simulink model "throttle_control"  (R2021a)
settings: Solver=FixedStepAuto  StartTime=0.0  StopTime=inf  FixedStep=1/2000  RelTol=1e-3
undefined symbols (not defined in the file): Brake, Steer, Throttle
libraries: robotlib x5, pid_lib x2
settings Model: Creator=refulgent  LastModifiedBy=refulgent
settings OptimizationCC: EnhancedBackFolding=on  PassReuseOutputArgsAs=Individual arguments  ZeroExternalMemoryAtStartup=off  ZeroInternalMemoryAtStartup=off  MaxStackSize=64  OptimizeBlockOrder=speed  DifferentSizesBufferReuse=on  EfficientTunableParamExpr=on
settings DebuggingCC: ParameterTunabilityLossMsg=error
settings HardwareCC: ProdBitPerPointer=32  ProdBitPerSizeT=32  ProdBitPerPtrDiffT=32  ProdLargestAtomicFloat=None  ProdIntDivRoundTo=Undefined  ProdEndianess=Unspecified  ProdWordSize=32  ProdHWDeviceType=Generic->Unspecified (assume 32-bit Generic)
settings SFSimCC: MATLABDynamicMemAlloc=off
settings RTWCC: SystemTargetFile=ert.tlc  HardwareBoard=Robot Operating System (ROS)  TLCOptions="-aInlineSetEventsForThisBaseRateFcn=TLC_FALSE -aSuppressMultiTaskScheduler=TLC_FALSE  -aRateBasedStepFcn=0"  TemplateMakefile=ert_default_tmf  Toolchain=Catkin  TargetLang=C++
settings CodeAppCC: ForceParamTrailComments=on  IgnoreCustomStorageClasses=off  OperatorAnnotations=on  SimulinkDataObjDesc=on  SFDataObjDesc=on  InsertBlockDesc=on
settings ERTTargetCC: SupportContinuousTime=on

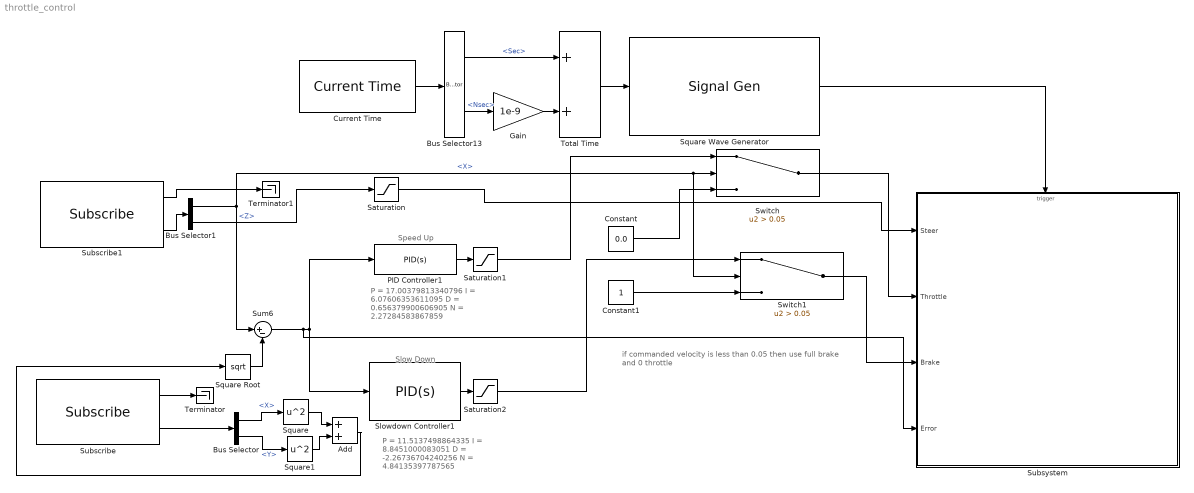
== system throttle_control ==
  note: if commanded velocity is less than 0.05 then use full brake
      | and 0 throttle
  note: P = 17.00379813340796
      | I = 6.07606353611095
      | D = 0.656379900606905
      | N = 2.27284583867859
  note: Slow Down
  note: Speed Up
  note: P = 11.5137498864335
      | I = 8.8451000083051
      | D = -2.26736704240256
      | N = 4.84135397787565
  Add : Sum
  Bus Selector : BusSelector  OutputSignals=Linear.X,Linear.Y
  Bus Selector1 : BusSelector  OutputSignals=Linear.X,Angular.Z
  Bus Selector13 : BusSelector  OutputSignals=Sec,Nsec
  Constant : Constant  Value=0.0
  Constant1 : Constant
  Current Time : robotlib/Current Time  OutputFormat=bus  SampleTime=-1  ModelName=throttle_control
      settings: SourceProductBaseCode=RR
  Gain : Gain  Gain=1e-9
  PID Controller1 : pid_lib/PID Controller  Controller=PID  Form=Parallel  TimeDomain=Continuous-time  UseExternalTs=off  SampleTime=-1  IntegratorMethod=Forward Euler  FilterMethod=Forward Euler  ControllerParametersSource=internal  P=17.00379813340796  I=6.07606353611095  D=0.656379900606905  UseFilter=on  N=2.27284583867859  TunerSelectOption=Transfer Function Based (PID Tuner App)  InitialConditionSource=internal  InitialConditionForIntegrator=0  InitialConditionForFilter=0  DifferentiatorICPrevScaledInput=0  ExternalReset=none  TrackingMode=off  Kt=1  LimitOutput=on  SatLimitsSource=internal  UpperSaturationLimit=1  LowerSaturationLimit=0  LinearizeAsGain=on  AntiWindupMode=clamping  Kb=1  POutMin=[]  POutMax=[]  IOutMin=[]  IOutMax=[]  DOutMin=[]  DOutMax=[]  NOutMin=[]  NOutMax=[]  SumOutMin=[]  SumOutMax=[]  SaturationOutMin=[]  SaturationOutMax=[]  PParamMin=[]  PParamMax=[]  IParamMin=[]  IParamMax=[]  DParamMin=[]  DParamMax=[]  NParamMin=[]  NParamMax=[]  KbParamMin=[]  KbParamMax=[]  KtParamMin=[]  KtParamMax=[]  KbOutMin=[]  KbOutMax=[]  KtOutMin=[]  KtOutMax=[]  IntegratorOutMin=[]  IntegratorOutMax=[]  FilterOutMin=[]  FilterOutMax=[]  SumI1OutMin=[]  SumI1OutMax=[]  SumI2OutMin=[]  SumI2OutMax=[]  SumI3OutMin=[]  SumI3OutMax=[]  SumI4OutMin=[]  SumI4OutMax=[]  SumDOutMin=[]  SumDOutMax=[]  DifferentiatorOutMin=[]  DifferentiatorOutMax=[]  FilterDiffOutCoefMin=[]  FilterDiffOutCoefMax=[]  ReciprocalOutMin=[]  ReciprocalOutMax=[]  SumDenOutMin=[]  SumDenOutMax=[]  SumNumOutMin=[]  SumNumOutMax=[]  DivideOutMin=[]  DivideOutMax=[]  UdiffTsProdOutMin=[]  UdiffTsProdOutMax=[]  NTsProdOutMin=[]  NTsProdOutMax=[]  UintegralTsProdOutMin=[]  UintegralTsProdOutMax=[]  UngainTsProdOutMin=[]  UngainTsProdOutMax=[]  IntegratorContinuousStateAttributes=''  IntegratorStateMustResolveToSignalObject=off  IntegratorRTWStateStorageClass=Auto  FilterContinuousStateAttributes=''  FilterStateMustResolveToSignalObject=off  FilterRTWStateStorageClass=Auto  ParallelPVariant=InternalParameters  IdealPVariant=Disabled  IVariant=InternalParameters  DVariant=InternalParameters  IntegratorVariant=Continuous  SatVariant=Enabled  AWVariant=ContClampingParallel  PCopyVariant=Disabled  TRVariant=Disabled  FdbkBlocksVariant=Forward  IdealPFdbkVariant=Disabled  SatFdbkVariant=Disabled  DerivativeFilterVariant=ContFilter  NVariant=InternalParameters  NCopyVariant=Disabled  FilterICVariant=InternalICsFilter  IntegratorICVariant=InternalICs  ExternalResetVariant=Disabled  TRSumVariant=Passthrough  SumFdbkVariant=Disabled  SumVariant=Sum_PID  TsampFilterVariant=InternalTs  TsampNgainVariant=Passthrough  TsampIntegralVariant=Passthrough  ExternalSaturationOutDataTypeStr=Inherit: Same as second input
  Saturation : Saturate  UpperLimit=1  LowerLimit=-1
  Saturation1 : Saturate  UpperLimit=1  LowerLimit=0
  Saturation2 : Saturate  UpperLimit=1  LowerLimit=0
  Slowdown Controller1 : pid_lib/PID Controller  Controller=PID  Form=Parallel  TimeDomain=Continuous-time  UseExternalTs=off  SampleTime=-1  IntegratorMethod=Forward Euler  FilterMethod=Forward Euler  ControllerParametersSource=internal  P=11.5137498864335  I=8.8451000083051  D=-2.26736704240256  UseFilter=on  N=4.84135397787565  TunerSelectOption=Transfer Function Based (PID Tuner App)  InitialConditionSource=internal  InitialConditionForIntegrator=0  InitialConditionForFilter=0  DifferentiatorICPrevScaledInput=0  ExternalReset=none  TrackingMode=off  Kt=1  LimitOutput=on  SatLimitsSource=internal  UpperSaturationLimit=1  LowerSaturationLimit=0  LinearizeAsGain=on  AntiWindupMode=clamping  Kb=1  POutMin=[]  POutMax=[]  IOutMin=[]  IOutMax=[]  DOutMin=[]  DOutMax=[]  NOutMin=[]  NOutMax=[]  SumOutMin=[]  SumOutMax=[]  SaturationOutMin=[]  SaturationOutMax=[]  PParamMin=[]  PParamMax=[]  IParamMin=[]  IParamMax=[]  DParamMin=[]  DParamMax=[]  NParamMin=[]  NParamMax=[]  KbParamMin=[]  KbParamMax=[]  KtParamMin=[]  KtParamMax=[]  KbOutMin=[]  KbOutMax=[]  KtOutMin=[]  KtOutMax=[]  IntegratorOutMin=[]  IntegratorOutMax=[]  FilterOutMin=[]  FilterOutMax=[]  SumI1OutMin=[]  SumI1OutMax=[]  SumI2OutMin=[]  SumI2OutMax=[]  SumI3OutMin=[]  SumI3OutMax=[]  SumI4OutMin=[]  SumI4OutMax=[]  SumDOutMin=[]  SumDOutMax=[]  DifferentiatorOutMin=[]  DifferentiatorOutMax=[]  FilterDiffOutCoefMin=[]  FilterDiffOutCoefMax=[]  ReciprocalOutMin=[]  ReciprocalOutMax=[]  SumDenOutMin=[]  SumDenOutMax=[]  SumNumOutMin=[]  SumNumOutMax=[]  DivideOutMin=[]  DivideOutMax=[]  UdiffTsProdOutMin=[]  UdiffTsProdOutMax=[]  NTsProdOutMin=[]  NTsProdOutMax=[]  UintegralTsProdOutMin=[]  UintegralTsProdOutMax=[]  UngainTsProdOutMin=[]  UngainTsProdOutMax=[]  IntegratorContinuousStateAttributes=''  IntegratorStateMustResolveToSignalObject=off  IntegratorRTWStateStorageClass=Auto  FilterContinuousStateAttributes=''  FilterStateMustResolveToSignalObject=off  FilterRTWStateStorageClass=Auto  ParallelPVariant=InternalParameters  IdealPVariant=Disabled  IVariant=InternalParameters  DVariant=InternalParameters  IntegratorVariant=Continuous  SatVariant=Enabled  AWVariant=ContClampingParallel  PCopyVariant=Disabled  TRVariant=Disabled  FdbkBlocksVariant=Forward  IdealPFdbkVariant=Disabled  SatFdbkVariant=Disabled  DerivativeFilterVariant=ContFilter  NVariant=InternalParameters  NCopyVariant=Disabled  FilterICVariant=InternalICsFilter  IntegratorICVariant=InternalICs  ExternalResetVariant=Disabled  TRSumVariant=Passthrough  SumFdbkVariant=Disabled  SumVariant=Sum_PID  TsampFilterVariant=InternalTs  TsampNgainVariant=Passthrough  TsampIntegralVariant=Passthrough  ExternalSaturationOutDataTypeStr=Inherit: Same as second input
  Square : Math  Operator=square  SaturateOnIntegerOverflow=on
  Square Root : Sqrt  SaturateOnIntegerOverflow=on
  Square Wave Generator : SignalGenerator  WaveForm=square  TimeSource=Use external signal  Frequency=100
  Square1 : Math  Operator=square  SaturateOnIntegerOverflow=on
  Subscribe : robotlib/Subscribe  topicSource=Specify your own  topic=vel  messageType=geometry_msgs/Twist  SampleTime=-1  legacyBusStruct=off  messageQueueLength=1
  Subscribe1 : robotlib/Subscribe  topicSource=Specify your own  topic=cmd_vel  messageType=geometry_msgs/Twist  SampleTime=-1  legacyBusStruct=off  messageQueueLength=1
  Subsystem : Subsystem
  Sum6 : Sum  Inputs=|+-
  Switch : Switch  Criteria=u2 > Threshold  Threshold=0.05
  Switch1 : Switch  Criteria=u2 > Threshold  Threshold=0.05
  Terminator : Terminator
  Terminator1 : Terminator
  Total Time : Sum
  wires:
  Sum6/1 -> Subsystem/4(Error), Slowdown Controller1/1, PID Controller1/1
  Subscribe/2 -> Bus Selector/1
  Bus Selector/1 -> Square/1  "<X>"
  Bus Selector/2 -> Square1/1  "<Y>"
  Square1/1 -> Add/2
  Square/1 -> Add/1
  Add/1 -> Square Root/1
  Square Root/1 -> Sum6/2
  Subscribe/1 -> Terminator/1
  Subscribe1/1 -> Terminator1/1
  Subscribe1/2 -> Bus Selector1/1
  Bus Selector1/1 -> Sum6/1, Switch1/2, Switch/2  "<X>"
  Bus Selector1/2 -> Saturation/1  "<Z>"
  Saturation/1 -> Subsystem/1(Steer)
  Saturation1/1 -> Switch/1
  Slowdown Controller1/1 -> Saturation2/1
  Bus Selector13/1 -> Total Time/1  "<Sec>"
  Square Wave Generator/1 -> Subsystem/Trigger
  Bus Selector13/2 -> Gain/1  "<Nsec>"
  Total Time/1 -> Square Wave Generator/1
  Gain/1 -> Total Time/2
  Current Time/1 -> Bus Selector13/1
  PID Controller1/1 -> Saturation1/1
  Saturation2/1 -> Switch1/1
  Constant/1 -> Switch/3
  Switch/1 -> Subsystem/2(Throttle)
  Constant1/1 -> Switch1/3
  Switch1/1 -> Subsystem/3(Brake)

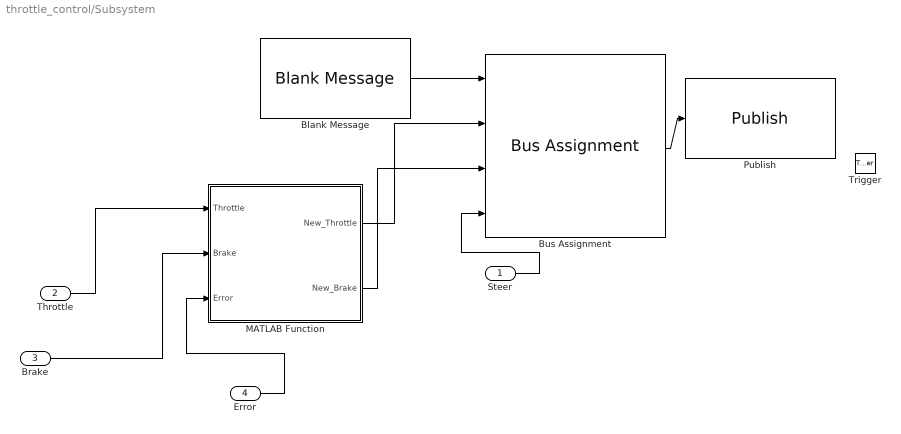
== system throttle_control/Subsystem ==
  Steer : Inport
  Throttle : Inport  Port=2
  Brake : Inport  Port=3
  Error : Inport  Port=4
  Trigger : TriggerPort  VariantControl=(inherit)  PortDimensions=1
  Blank Message : robotlib/Blank Message  messageClass=Message  entityType=steer/avcontrol  messageType=steer/avcontrol  SampleTime=inf  legacyBusStruct=off
  Bus Assignment : BusAssignment  AssignedSignals=Throttle,Brake,Steer
  MATLAB Function : MATLAB Function  TreatAsAtomicUnit=on
  Publish : robotlib/Publish  topicSource=Specify your own  topic=control  messageType=steer/avcontrol  legacyBusStruct=off  messageQueueLength=1
  wires:
  Bus Assignment/1 -> Publish/1
  Blank Message/1 -> Bus Assignment/1
  Throttle/1 -> MATLAB Function/1(Throttle)
  Brake/1 -> MATLAB Function/2(Brake)
  Steer/1 -> Bus Assignment/4
  Error/1 -> MATLAB Function/3(Error)
  MATLAB Function/1(New_Throttle) -> Bus Assignment/2
  MATLAB Function/2(New_Brake) -> Bus Assignment/3

== matlab function throttle_control/Subsystem/MATLAB Function ==
  data: Throttle input; New_Throttle output; Brake input; Error input; New_Brake output
function [New_Throttle, New_Brake] = fcn(Throttle, Brake, Error)

    New_Throttle = Throttle;
    New_Brake= Brake;

    if(Throttle == Brake)
        % Commanded velocity is greater than current velocity then accelerate
        if (Error >= 0)
            New_Throttle = Throttle;
            New_Brake = 0;
        elseif(Error < 0)
            New_Throttle = 0.0;
            New_Brake = Brake;
        end
    end
end
